simulink model "q14"  (R2019a)
settings: Solver=FixedStepAuto  StartTime=0.0  StopTime=0.1  FixedStep=1e-7  RelTol=1e-3
libraries: simulink x2
settings Model: Creator=marco  LastModifiedBy=marco

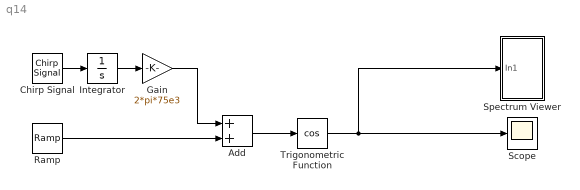
== system q14 ==
  Add : Sum
  Chirp Signal : simulink/Sources/Chirp Signal  f1=100  T=0.1  f2=4000
  Gain : Gain  Gain=2*pi*75e3
  Integrator : Integrator
  Ramp : simulink/Sources/Ramp  slope=2*pi*(1e6)  start=0  InitialOutput=0
  Scope : Scope
  Spectrum Viewer : Subsystem
  Trigonometric Function : Trigonometry  Operator=cos
  wires:
  Add/1 -> Trigonometric Function/1
  Trigonometric Function/1 -> Spectrum Viewer/1(In1), Scope/1
  Ramp/1 -> Add/2
  Chirp Signal/1 -> Integrator/1
  Integrator/1 -> Gain/1
  Gain/1 -> Add/1

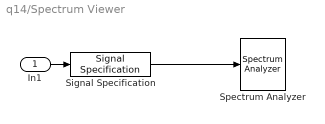
== system q14/Spectrum Viewer ==
  In1 : Inport
  Signal Specification : SignalSpecification  SampleTime=1e-7
  Spectrum Analyzer : SpectrumAnalyzer
  wires:
  In1/1 -> Signal Specification/1
  Signal Specification/1 -> Spectrum Analyzer/1
